simulink model "water_network_sim"  (R2013b)
settings: Solver=ode45  StartTime=0.0  StopTime=80  RelTol=1e-3
values from neighbouring files (symbols this model uses):
  Cd = [0.01 Ti 0]    [water_network_sim_init.m]
  Cn = [Kp*Ti*Td Ti 1]    [water_network_sim_init.m]
  H1d = [tp 1]    [water_network_sim_init.m]
  H1n = [kp]    [water_network_sim_init.m]
  H2d = [tp 1]    [water_network_sim_init.m]
  H2n = [kp]    [water_network_sim_init.m]
  H3d = [tp 1]    [water_network_sim_init.m]
  H3n = [kp]    [water_network_sim_init.m]
  H4d = [tp 1]    [water_network_sim_init.m]
  H4n = [kp]    [water_network_sim_init.m]
settings Model: Creator=alex  LastModifiedBy=alex

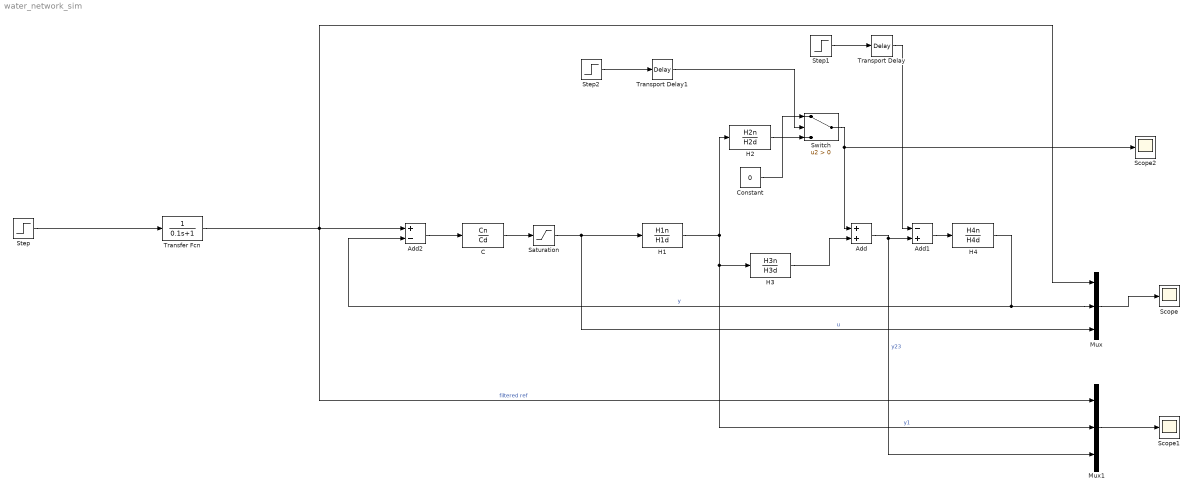
== system water_network_sim ==
  Add : Sum
  Add1 : Sum  Inputs=-+
  Add2 : Sum  Inputs=+-
  "C " : TransferFcn  Numerator=Cn  Denominator=Cd
  Constant : Constant  Value=0
  H1 : TransferFcn  Numerator=H1n  Denominator=H1d
  H2 : TransferFcn  Numerator=H2n  Denominator=H2d
  H3 : TransferFcn  Numerator=H3n  Denominator=H3d
  H4 : TransferFcn  Numerator=H4n  Denominator=H4d
  Mux : Mux  Inputs=3
  Mux1 : Mux  Inputs=3
  Saturation : Saturate  UpperLimit=20  LowerLimit=0
  Scope : Scope
      settings: ShowLegends=on
  Scope1 : Scope
      settings: ShowLegends=on
  Scope2 : Scope
      settings: SaveName=ScopeData2
  Step : Step  SampleTime=0
  Step1 : Step  SampleTime=0
  Step2 : Step  SampleTime=0
  Switch : Switch  Criteria=u2 > Threshold
  Transfer Fcn : TransferFcn  Denominator=[0.1 1]
  Transport Delay : TransportDelay  DelayTime=35
  Transport Delay1 : TransportDelay  DelayTime=45
  wires:
  H1/1 -> Mux1/2, H3/1, H2/1  "y1"
  H3/1 -> Add/2
  Add/1 -> Add1/2, Mux1/3  "y23"
  Mux/1 -> Scope/1
  Mux1/1 -> Scope1/1
  H4/1 -> Mux/2, Add2/2  "y"
  Add1/1 -> H4/1
  Step1/1 -> Transport Delay/1
  Transport Delay/1 -> Add1/1
  "C "/1 -> Saturation/1
  Add2/1 -> "C "/1
  Step/1 -> Transfer Fcn/1
  Saturation/1 -> Mux/3, H1/1  "u"
  Transfer Fcn/1 -> Mux1/1, Mux/1, Add2/1  "filtered ref"
  Switch/1 -> Scope2/1, Add/1
  Step2/1 -> Transport Delay1/1
  Transport Delay1/1 -> Switch/2
  Constant/1 -> Switch/1
  H2/1 -> Switch/3
